simulink model "qpskTest"  (R2019b)
settings: Solver=VariableStepAuto  StartTime=0.0  StopTime=0.08  RelTol=1e-3
undefined symbols (not defined in the file): doppler, rsgenpoly
libraries: dspobslib x46, dspindex x4, commdigbbndpm3 x4, commchan3 x2, dspxfrm3 x2, commblkcod2 x2, commseqgen2 x2, commutil2 x2, commrandsrc2 x1, dspsigops x1, commsink2 x1
settings Model: Creator=mgege007  LastModifiedBy=mgege007

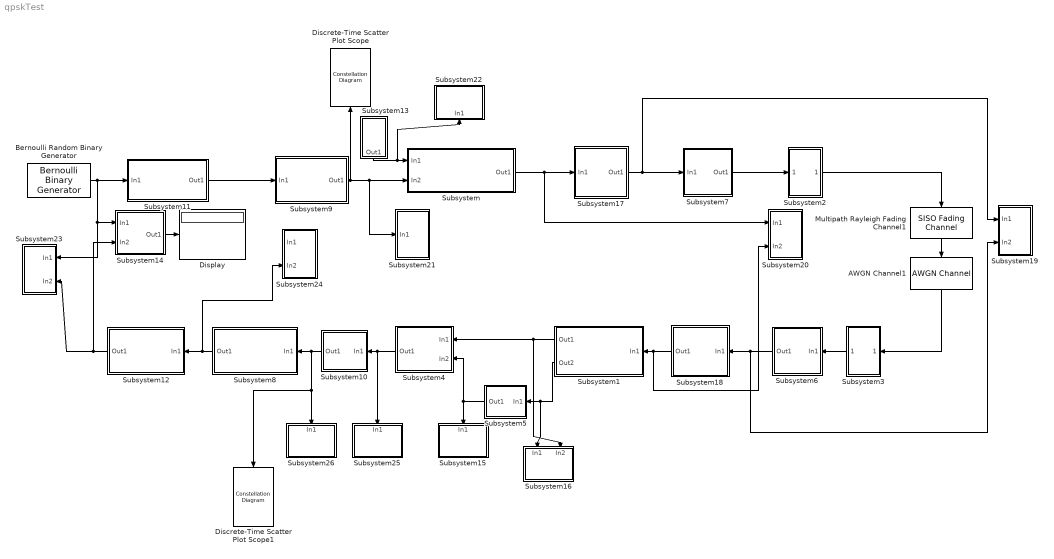
== system qpskTest ==
  AWGN Channel1 : commchan3/AWGN Channel  InputProcessing=Columns as channels (frame based)  seed=32965  noiseMode="Signal to noise ratio  (SNR)"  EbNodB=10  EsNodB=28  SNRdB=-15  bitsPerSym=1  Ps=30/(5.5e5*11/15*2.4)*1.08  Tsym=80e-6  variance=1
      settings: SourceProductName=Communications Toolbox
  Bernoulli Random Binary Generator : commrandsrc2/Bernoulli Binary Generator  P=[0.5]  seed=9364248  Ts=16e-5/44/2  frameBased=on  sampPerFrame=44  orient=off  outDataType=double
      settings: SourceProductName=Communications Toolbox  SourceProductBaseCode=CM
  Discrete-Time Scatter Plot Scope : ConstellationDiagram  Tag=ScatterPlot
  Discrete-Time Scatter Plot Scope1 : ConstellationDiagram  Tag=ScatterPlot
  Display : Display
  Multipath Rayleigh Fading Channel1 : commchan3/SISO Fading Channel  InheritSampleRate=on  SampleRate=1  PathDelays=[0 2e-6]  AveragePathGains=[0 -12]  NormalizePathGains=on  FadingDistribution=Rayleigh  KFactor=3  DirectPathDopplerShift=0  DirectPathInitialPhase=0  MaximumDopplerShift=40  DopplerSpectrum=doppler('Jakes')  RandomStream=mt19937ar with seed  Seed=73  PathGainsOutputPort=off  ChannelFilterDelayOutputPort=off  SimulateUsing=Interpreted execution  Visualization=Off  PathsForDopplerDisplay=1  SamplesToDisplay=25%
      settings: SourceProductName=Communications Toolbox
  Subsystem : Subsystem
      mask Display: disp('OFDM Baseband\nModulator\ndan\nAdd Cyclic Prefix')
  Subsystem1 : Subsystem
      mask Display: disp('OFDM Baseband\nDemodulator\ndan \nRemove Cyclic prefix')
  Subsystem10 : Subsystem
      mask Display: disp('Remove\nZero')
  Subsystem11 : Subsystem
      mask Display: disp('RS(15,11) Encoder')
  Subsystem12 : Subsystem
      mask Display: disp('RS(15,11) Decoder')
  Subsystem13 : Subsystem
      mask Display: disp('Training')
  Subsystem14 : Subsystem
      mask Display: disp('SER\nCalculation')
  Subsystem15 : Subsystem
  Subsystem16 : Subsystem
  Subsystem17 : Subsystem
      mask Display: disp('Add\nCyclic Prefix')
  Subsystem18 : Subsystem
      mask Display: disp('Remove\nCyclic Prefix')
  Subsystem19 : Subsystem
  Subsystem2 : Subsystem
      mask Display: disp('P/S')
  Subsystem20 : Subsystem
  Subsystem21 : Subsystem
  Subsystem22 : Subsystem
  Subsystem23 : Subsystem
  Subsystem24 : Subsystem
  Subsystem25 : Subsystem
  Subsystem26 : Subsystem
  Subsystem3 : Subsystem
      mask Display: disp('S/P')
  Subsystem4 : Subsystem
      mask Display: disp('Channel\nCompensation')
  Subsystem5 : Subsystem
      mask Display: disp('Channel\nEstimator')
  Subsystem6 : Subsystem
      mask Display: disp('Training\nSeparation')
  Subsystem7 : Subsystem
      mask Display: disp('Training\nInsertion')
  Subsystem8 : Subsystem
      mask Display: disp('QPSK Demapping')
  Subsystem9 : Subsystem
      mask Display: disp('QPSK Mapping')
  wires:
  Subsystem3/1(Out1) -> Subsystem6/1(In1)
  Subsystem17/1(Out1) -> Subsystem7/1(In1), Subsystem19/1(In1)
  Subsystem11/1(Out1) -> Subsystem9/1(In1)
  Subsystem13/1(Out1) -> Subsystem/1(In1), Subsystem22/1(In1)
  Subsystem6/1(Out1) -> Subsystem18/1(In1), Subsystem19/2(In2)
  Subsystem10/1(Out1) -> Subsystem8/1(In1), Subsystem26/1(In1), Discrete-Time Scatter Plot Scope1/1
  Bernoulli Random Binary Generator/1 -> Subsystem14/1(In1), Subsystem23/1(In1), Subsystem11/1(In1)
  Subsystem2/1(Out1) -> Multipath Rayleigh Fading Channel1/1
  Subsystem18/1(Out1) -> Subsystem1/1(In1), Subsystem20/2(In2)
  Subsystem14/1(Out1) -> Display/1
  Subsystem1/1(Out1) -> Subsystem4/1(In1), Subsystem16/2(In2)
  Multipath Rayleigh Fading Channel1/1 -> AWGN Channel1/1
  AWGN Channel1/1 -> Subsystem3/1(In1)
  Subsystem4/1(Out1) -> Subsystem10/1(In1), Subsystem25/1(In1)
  Subsystem7/1(Out1) -> Subsystem2/1(In1)
  Subsystem9/1(Out1) -> Subsystem/2(In2), Subsystem21/1(In1), Discrete-Time Scatter Plot Scope/1
  Subsystem5/1(Out1) -> Subsystem4/2(In2), Subsystem15/1(In1)
  Subsystem12/1(Out1) -> Subsystem14/2(In2), Subsystem23/2(In2)
  Subsystem1/2(Out2) -> Subsystem5/1(In1), Subsystem16/1(In1)
  Subsystem8/1(Out1) -> Subsystem12/1(In1), Subsystem24/2(In2)
  Subsystem/1(Out1) -> Subsystem17/1(In1), Subsystem20/1(In1)

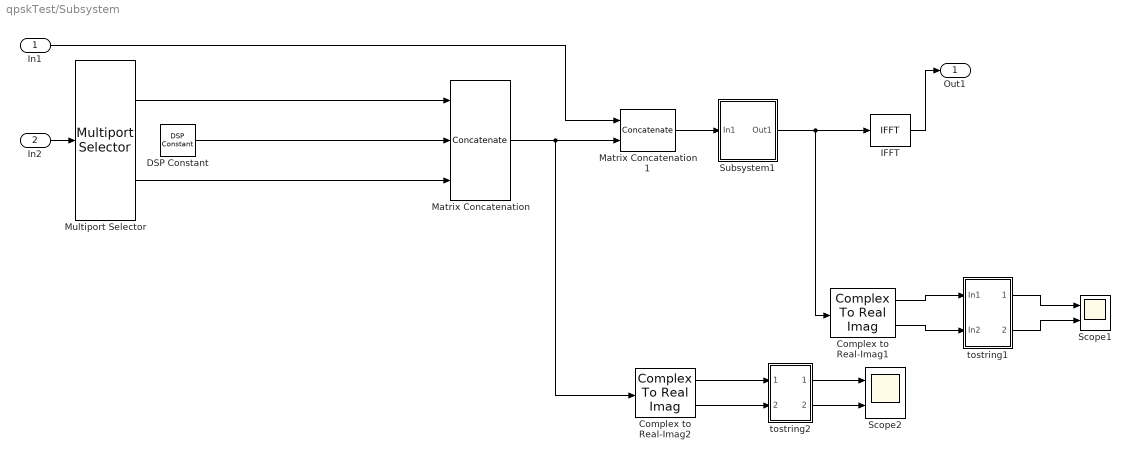
== system qpskTest/Subsystem ==
  In1 : Inport
  In2 : Inport  Port=2
  Complex to Real-Imag1 : ComplexToRealImag
  Complex to Real-Imag2 : ComplexToRealImag
  DSP Constant : dspobslib/DSP Constant  Value=0  SampleMode=Discrete  discreteOutput=Frame-based  continuousOutput=Sample-based  sampTime=16e-5/2  framePeriod=16e-5/2  dataType=Inherit from 'Constant value'  isSigned=on  wordLen=16  udDataType=sfix(16)  fracBitsMode=Best precision  numFracBits=15  InterpretAs1D=off  Ts=16e-5/2  FramebasedOutput=on
      settings: SourceProductName=DSP System Toolbox  SourceProductBaseCode=DS
  IFFT : dspxfrm3/IFFT  FFTImplementation=Auto  CompMethod=Table lookup  TableOpt=HYBRID  TableOptActive=Speed  BitRevOrder=off  cs_in=off  Normalize=on  InheritFFTLength=on  FFTLength=64  WrapInput=on  mode=Real  outSamplingMode=Frame based  roundingMode=Floor  overflowMode=off  firstCoeffDataTypeStr=Inherit: Same word length as input  firstCoeffLastDataTypeStr=Inherit: Same word length as input  outputMin=[]  outputMax=[]
      settings: SourceProductName=DSP System Toolbox
  Matrix Concatenation : Concatenate  NumInputs=3  Mode=Multidimensional array
  Matrix Concatenation1 : Concatenate  Mode=Multidimensional array  ConcatenateDimension=2
  Multiport Selector : dspindex/Multiport Selector  rowsOrCols=Rows  idxCellArray={1:15,16:30}  idxErrMode=Clip Index
  Scope1 : Scope  NumInputPorts=2
  Scope2 : Scope  NumInputPorts=2
  Subsystem1 : Subsystem
      mask Display: disp('Zero Pad')
  tostring1 : Subsystem
  tostring2 : Subsystem
  Out1 : Outport
  wires:
  IFFT/1 -> Out1/1
  Multiport Selector/1 -> Matrix Concatenation/1
  Multiport Selector/2 -> Matrix Concatenation/3
  DSP Constant/1 -> Matrix Concatenation/2
  Subsystem1/1(Out1) -> IFFT/1, Complex to Real-Imag1/1
  In2/1 -> Multiport Selector/1
  Matrix Concatenation1/1 -> Subsystem1/1(In1)
  Matrix Concatenation/1 -> Matrix Concatenation1/2, Complex to Real-Imag2/1
  In1/1 -> Matrix Concatenation1/1
  Complex to Real-Imag1/1 -> tostring1/1(In1)
  Complex to Real-Imag1/2 -> tostring1/2(In2)
  tostring1/1(Out1) -> Scope1/1
  tostring1/2(Out2) -> Scope1/2
  Complex to Real-Imag2/1 -> tostring2/1(In1)
  Complex to Real-Imag2/2 -> tostring2/2(In2)
  tostring2/1(Out1) -> Scope2/1
  tostring2/2(Out2) -> Scope2/2

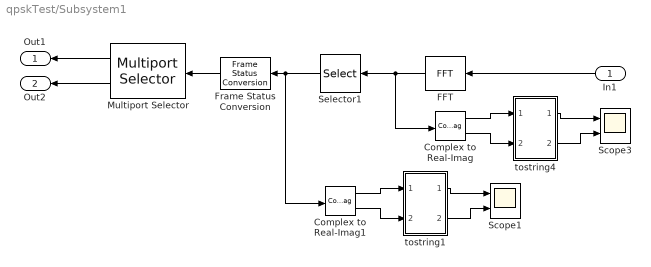
== system qpskTest/Subsystem1 ==
  In1 : Inport
  Complex to Real-Imag : ComplexToRealImag
  Complex to Real-Imag1 : ComplexToRealImag
  FFT : dspxfrm3/FFT  FFTImplementation=Auto  CompMethod=Table lookup  TableOpt=HYBRID  TableOptActive=Speed  BitRevOrder=off  Normalize=off  InheritFFTLength=on  FFTLength=64  WrapInput=on  roundingMode=Floor  overflowMode=off  firstCoeffDataTypeStr=Inherit: Same word length as input  firstCoeffLastDataTypeStr=Inherit: Same word length as input  outputMin=[]  outputMax=[]
  Frame Status Conversion : dspobslib/Frame Status Conversion  growRefPort=off  outframe=Frame-based
      settings: SourceProductName=DSP System Toolbox  SourceProductBaseCode=DS
  Multiport Selector : dspindex/Multiport Selector  rowsOrCols=Columns  idxCellArray={1,2}  idxErrMode=Clip Index
  Scope1 : Scope  NumInputPorts=2
  Scope3 : Scope  NumInputPorts=2
  Selector1 : Selector  NumberOfDimensions=2  InputPortWidth=64  IndexOptions=Index vector (dialog),Select all  Indices=[50:64,1:16],-1  OutputSizes=1
  tostring1 : Subsystem
  tostring4 : Subsystem
  Out1 : Outport
  Out2 : Outport  Port=2
  wires:
  FFT/1 -> Selector1/1, Complex to Real-Imag/1
  Selector1/1 -> Frame Status Conversion/1, Complex to Real-Imag1/1
  In1/1 -> FFT/1
  Frame Status Conversion/1 -> Multiport Selector/1
  Multiport Selector/1 -> Out1/1
  Multiport Selector/2 -> Out2/1
  Complex to Real-Imag/1 -> tostring4/1(In1)
  Complex to Real-Imag/2 -> tostring4/2(In2)
  tostring4/1(Out1) -> Scope3/1
  tostring4/2(Out2) -> Scope3/2
  Complex to Real-Imag1/1 -> tostring1/1(In1)
  Complex to Real-Imag1/2 -> tostring1/2(In2)
  tostring1/1(Out1) -> Scope1/1
  tostring1/2(Out2) -> Scope1/2

== system qpskTest/Subsystem10 ==
  In1 : Inport
  Selector2 : Selector  NumberOfDimensions=2  InputPortWidth=31  IndexOptions=Index vector (dialog),Select all  Indices=[1:15,17:31],-1  OutputSizes=1
  Out1 : Outport
  wires:
  Selector2/1 -> Out1/1
  In1/1 -> Selector2/1

== system qpskTest/Subsystem11 ==
  In1 : Inport
  Binary-Input RS Encoder : commblkcod2/Binary-Input RS Encoder  n=15  k=11  specShortening=off  shortenedK=3  specGenPoly=off  genPoly=rsgenpoly(7,3)  specPrimPoly=off  prPoly=[1 0 1 1]  specPuncture=off  punctVec=[ones(2,1); zeros(2,1)]  outDType=Same as input
      settings: SourceProductName=Communications Toolbox  SourceProductBaseCode=CM
  Out1 : Outport
  wires:
  In1/1 -> Binary-Input RS Encoder/1
  Binary-Input RS Encoder/1 -> Out1/1

== system qpskTest/Subsystem12 ==
  In1 : Inport
  Binary-Output RS Decoder : commblkcod2/Binary-Output RS Decoder  n=15  k=11  specShortening=off  shortenedK=3  specGenPoly=off  genPoly=rsgenpoly(7,3)  specPrimPoly=off  prPoly=[1 0 1 1]  specPuncture=off  punctVec=[ones(2,1); zeros(2,1)]  specErasurePort=off  showNumErr=on  outDType=Same as input
      settings: SourceProductName=Communications Toolbox  SourceProductBaseCode=CM
  Terminator : Terminator
  Out1 : Outport
  wires:
  Binary-Output RS Decoder/2 -> Terminator/1
  Binary-Output RS Decoder/1 -> Out1/1
  In1/1 -> Binary-Output RS Decoder/1

== system qpskTest/Subsystem13 ==
  PN Sequence Generator : commseqgen2/PN Sequence Generator  poly=[1 0 0 0 0 1 1]  ini_sta=[0 0 0 0 0 1]  outBitMaskSource=Dialog parameter  shift=0  outVarSiz=off  maxOutSizeMode=Dialog parameter  maxOutSize=[10 1]  Ts=16e-5/2/31  frameBased=on  sampPerFrame=31  reset=off  bitPackedOutputs=off  outDataType=double  numPackedBits=8  bitPackDataSigned=off  bitPackedOutDType=double
      settings: SourceProductName=Communications Toolbox  SourceProductBaseCode=CM
  Unipolar to Bipolar Converter : commutil2/Unipolar to Bipolar Converter  M=2  polarity=Positive  dataType=Inherit via internal rule
      settings: SourceProductName=Communications Toolbox
  Out1 : Outport
  wires:
  PN Sequence Generator/1 -> Unipolar to Bipolar Converter/1
  Unipolar to Bipolar Converter/1 -> Out1/1

== system qpskTest/Subsystem14 ==
  In1 : Inport
  In2 : Inport  Port=2
  Error Rate Calculation : commsink2/Error Rate Calculation  N=22  st_delay=0  cp_mode=Entire frame  subframe=[]  PMode=Port  WsName=ErrorVec  RsMode2=off  stop=off  numErr=inf  maxBits=2e4
      settings: SourceProductName=Communications Toolbox
  QPSK Modulator Baseband : commdigbbndpm3/QPSK Modulator Baseband  InType=Bit  Enc=Binary  Ph=pi/4  outDtype=double  outWordLen=16  outUDDataType=sfix(16)  outFracLenMode=Best precision  outFracLen=15  outDataTypeStr=double  outLastDataTypeStr=double
      settings: SourceProductName=Communications Toolbox
  QPSK Modulator Baseband1 : commdigbbndpm3/QPSK Modulator Baseband  InType=Bit  Enc=Binary  Ph=pi/4  outDtype=double  outWordLen=16  outUDDataType=sfix(16)  outFracLenMode=Best precision  outFracLen=15  outDataTypeStr=double  outLastDataTypeStr=double
      settings: SourceProductName=Communications Toolbox
  Out1 : Outport
  wires:
  QPSK Modulator Baseband/1 -> Error Rate Calculation/1
  QPSK Modulator Baseband1/1 -> Error Rate Calculation/2
  In1/1 -> QPSK Modulator Baseband/1
  Error Rate Calculation/1 -> Out1/1
  In2/1 -> QPSK Modulator Baseband1/1

== system qpskTest/Subsystem15 ==
  In1 : Inport
  Complex to Real-Imag7 : ComplexToRealImag
  Scope7 : Scope  NumInputPorts=2
  tostring9 : Subsystem
  wires:
  Complex to Real-Imag7/1 -> tostring9/1(In1)
  Complex to Real-Imag7/2 -> tostring9/2(In2)
  tostring9/1(Out1) -> Scope7/1
  tostring9/2(Out2) -> Scope7/2
  In1/1 -> Complex to Real-Imag7/1

== system qpskTest/Subsystem16 ==
  In1 : Inport
  In2 : Inport  Port=2
  Complex to Real-Imag5 : ComplexToRealImag
  Complex to Real-Imag6 : ComplexToRealImag
  Scope6 : Scope  NumInputPorts=4
  tostring8 : Subsystem
  wires:
  tostring8/1(Out1) -> Scope6/1
  tostring8/2(Out2) -> Scope6/2
  Complex to Real-Imag5/1 -> tostring8/1(In1)
  Complex to Real-Imag5/2 -> tostring8/2(In2)
  Complex to Real-Imag6/1 -> tostring8/3(In3)
  Complex to Real-Imag6/2 -> tostring8/4(In4)
  tostring8/3(Out3) -> Scope6/3
  tostring8/4(Out4) -> Scope6/4
  In1/1 -> Complex to Real-Imag5/1
  In2/1 -> Complex to Real-Imag6/1

== system qpskTest/Subsystem17 ==
  In1 : Inport
  Selector3 : Selector  NumberOfDimensions=2  InputPortWidth=64  IndexOptions=Index vector (dialog),Select all  Indices=[39:64,1:64],-1  OutputSizes=1
  Out1 : Outport
  wires:
  Selector3/1 -> Out1/1
  In1/1 -> Selector3/1

== system qpskTest/Subsystem18 ==
  In1 : Inport
  Selector4 : Selector  NumberOfDimensions=2  InputPortWidth=78  IndexOptions=Index vector (dialog),Select all  Indices=[27:90],-1  OutputSizes=1
  Out1 : Outport
  wires:
  Selector4/1 -> Out1/1
  In1/1 -> Selector4/1

== system qpskTest/Subsystem19 ==
  In1 : Inport
  In2 : Inport  Port=2
  Complex to Real-Imag1 : ComplexToRealImag
  Complex to Real-Imag2 : ComplexToRealImag
  Scope4 : Scope  NumInputPorts=4
  tostring5 : Subsystem
  tostring6 : Subsystem
  wires:
  Complex to Real-Imag1/1 -> tostring5/1(In1)
  Complex to Real-Imag1/2 -> tostring5/2(In2)
  tostring5/1(Out1) -> Scope4/1
  Complex to Real-Imag2/1 -> tostring6/1(In1)
  Complex to Real-Imag2/2 -> tostring6/2(In2)
  tostring6/1(Out1) -> Scope4/2
  tostring5/2(Out2) -> Scope4/3
  tostring6/2(Out2) -> Scope4/4
  In1/1 -> Complex to Real-Imag1/1
  In2/1 -> Complex to Real-Imag2/1

== system qpskTest/Subsystem2 ==
  In1 : Inport
  Unbuffer3 : Unbuffer
  Out1 : Outport
  wires:
  In1/1 -> Unbuffer3/1
  Unbuffer3/1 -> Out1/1

== system qpskTest/Subsystem20 ==
  In1 : Inport
  In2 : Inport  Port=2
  Complex to Real-Imag3 : ComplexToRealImag
  Complex to Real-Imag4 : ComplexToRealImag
  Scope5 : Scope  NumInputPorts=4
  tostring7 : Subsystem
  wires:
  Complex to Real-Imag3/1 -> tostring7/1(In1)
  Complex to Real-Imag3/2 -> tostring7/2(In2)
  tostring7/1(Out1) -> Scope5/1
  Complex to Real-Imag4/1 -> tostring7/3(In3)
  Complex to Real-Imag4/2 -> tostring7/4(In4)
  tostring7/3(Out3) -> Scope5/2
  tostring7/2(Out2) -> Scope5/3
  tostring7/4(Out4) -> Scope5/4
  In1/1 -> Complex to Real-Imag3/1
  In2/1 -> Complex to Real-Imag4/1

== system qpskTest/Subsystem21 ==
  In1 : Inport
  Complex to Real-Imag : ComplexToRealImag
  Scope3 : Scope  NumInputPorts=2
  tostring4 : Subsystem
  wires:
  Complex to Real-Imag/1 -> tostring4/1(In1)
  Complex to Real-Imag/2 -> tostring4/2(In2)
  tostring4/1(Out1) -> Scope3/1
  tostring4/2(Out2) -> Scope3/2
  In1/1 -> Complex to Real-Imag/1

== system qpskTest/Subsystem22 ==
  In1 : Inport
  Scope2 : Scope
  tostring3 : Subsystem
  wires:
  tostring3/1(Out1) -> Scope2/1
  In1/1 -> tostring3/1(In1)

== system qpskTest/Subsystem23 ==
  In1 : Inport
  In2 : Inport  Port=2
  Scope : Scope  NumInputPorts=2
  tostring : Subsystem
  tostring1 : Subsystem
  wires:
  tostring/1(Out1) -> Scope/1
  tostring1/1(Out1) -> Scope/2
  In1/1 -> tostring/1(In1)
  In2/1 -> tostring1/1(In1)

== system qpskTest/Subsystem24 ==
  In1 : Inport
  In2 : Inport  Port=2
  Scope1 : Scope  NumInputPorts=2
  tostring2 : Subsystem
  wires:
  tostring2/1(Out1) -> Scope1/1
  tostring2/2(Out2) -> Scope1/2
  In1/1 -> tostring2/1(In1)
  In2/1 -> tostring2/2(In2)

== system qpskTest/Subsystem25 ==
  In1 : Inport
  Complex to Real-Imag7 : ComplexToRealImag
  Scope7 : Scope  NumInputPorts=2
  tostring9 : Subsystem
  wires:
  Complex to Real-Imag7/1 -> tostring9/1(In1)
  Complex to Real-Imag7/2 -> tostring9/2(In2)
  tostring9/1(Out1) -> Scope7/1
  tostring9/2(Out2) -> Scope7/2
  In1/1 -> Complex to Real-Imag7/1

== system qpskTest/Subsystem26 ==
  In1 : Inport
  Complex to Real-Imag7 : ComplexToRealImag
  Scope7 : Scope  NumInputPorts=2
  tostring9 : Subsystem
  wires:
  Complex to Real-Imag7/1 -> tostring9/1(In1)
  Complex to Real-Imag7/2 -> tostring9/2(In2)
  tostring9/1(Out1) -> Scope7/1
  tostring9/2(Out2) -> Scope7/2
  In1/1 -> Complex to Real-Imag7/1

== system qpskTest/Subsystem3 ==
  In1 : Inport
  Buffer : Buffer  N=180
  Out1 : Outport
  wires:
  In1/1 -> Buffer/1
  Buffer/1 -> Out1/1

== system qpskTest/Subsystem4 ==
  In1 : Inport
  In2 : Inport  Port=2
  Frame Status Conversion5 : dspobslib/Frame Status Conversion  growRefPort=off  outframe=Frame-based
      settings: SourceProductName=DSP System Toolbox  SourceProductBaseCode=DS
  Product : Product  SaturateOnIntegerOverflow=on  OutDataTypeStr=Inherit: Same as first input
  Out1 : Outport
  wires:
  Frame Status Conversion5/1 -> Out1/1
  In2/1 -> Product/1
  Product/1 -> Frame Status Conversion5/1
  In1/1 -> Product/2

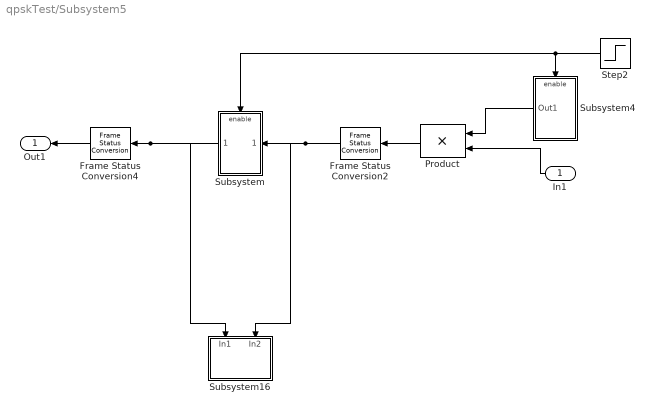
== system qpskTest/Subsystem5 ==
  In1 : Inport
  Frame Status Conversion2 : dspobslib/Frame Status Conversion  growRefPort=off  outframe=Frame-based
      settings: SourceProductName=DSP System Toolbox  SourceProductBaseCode=DS
  Frame Status Conversion4 : dspobslib/Frame Status Conversion  growRefPort=off  outframe=Frame-based
      settings: SourceProductName=DSP System Toolbox  SourceProductBaseCode=DS
  Product : Product  SaturateOnIntegerOverflow=on  OutDataTypeStr=Inherit: Same as first input
  Step2 : Step  Time=16e-5/2  SampleTime=16e-5/2
  Subsystem : Subsystem
  Subsystem16 : Subsystem
  Subsystem4 : Subsystem  TreatAsAtomicUnit=on
  Out1 : Outport
  wires:
  Step2/1 -> Subsystem4/Enable, Subsystem/Enable
  Subsystem4/1(Out1) -> Product/1
  Product/1 -> Frame Status Conversion2/1
  Frame Status Conversion2/1 -> Subsystem/1(In1), Subsystem16/2(In2)
  Frame Status Conversion4/1 -> Out1/1
  In1/1 -> Product/2
  Subsystem/1(Out1) -> Frame Status Conversion4/1, Subsystem16/1(In1)

== system qpskTest/Subsystem6 ==
  In1 : Inport
  Matrix Concatenation1 : Concatenate  Mode=Multidimensional array  ConcatenateDimension=2
  Multiport Selector1 : dspindex/Multiport Selector  rowsOrCols=Rows  idxCellArray={91:180,1:90}  idxErrMode=Clip Index
  Out1 : Outport
  wires:
  Multiport Selector1/2 -> Matrix Concatenation1/2
  Multiport Selector1/1 -> Matrix Concatenation1/1
  In1/1 -> Multiport Selector1/1
  Matrix Concatenation1/1 -> Out1/1

== system qpskTest/Subsystem7 ==
  In1 : Inport
  Frame Status Conversion : dspobslib/Frame Status Conversion  growRefPort=off  outframe=Frame-based
      settings: SourceProductName=DSP System Toolbox  SourceProductBaseCode=DS
  Matrix Concatenation : Concatenate  Mode=Multidimensional array
  Multiport Selector : dspindex/Multiport Selector  rowsOrCols=Columns  idxCellArray={1,2}  idxErrMode=Clip Index
  Out1 : Outport
  wires:
  Multiport Selector/1 -> Matrix Concatenation/1
  Multiport Selector/2 -> Matrix Concatenation/2
  Matrix Concatenation/1 -> Frame Status Conversion/1
  In1/1 -> Multiport Selector/1
  Frame Status Conversion/1 -> Out1/1

== system qpskTest/Subsystem8 ==
  In1 : Inport
  Gain : Gain  Gain=0.75  SaturateOnIntegerOverflow=on  OutDataTypeStr=Inherit: Same as input  ParamDataTypeStr=Inherit: Same as input
  QPSK Demodulator Baseband : commdigbbndpm3/QPSK Demodulator Baseband  OutType=Bit  DecType=Hard decision  VarSource=Dialog  Variance=1  Dec=Binary  Ph=pi/4  outDtype1=Inherit via internal rule  outDtype2=Inherit via internal rule  derotateFactorWordLen=16  derotateFactorDataTypeStr=Inherit: Same word length as input  derotateFactorLastDataTypeStr=Inherit: Same word length as input
      settings: SourceProductName=Communications Toolbox
  Rounding Function : Rounding  Operator=round
  Out1 : Outport
  wires:
  In1/1 -> Gain/1
  Rounding Function/1 -> Out1/1
  QPSK Demodulator Baseband/1 -> Rounding Function/1
  Gain/1 -> QPSK Demodulator Baseband/1

== system qpskTest/Subsystem9 ==
  In1 : Inport
  Gain : Gain  Gain=1/0.75  SaturateOnIntegerOverflow=on  OutDataTypeStr=Inherit: Same as input  ParamDataTypeStr=Inherit: Same as input
  QPSK Modulator Baseband : commdigbbndpm3/QPSK Modulator Baseband  InType=Bit  Enc=Binary  Ph=pi/4  outDtype=double  outWordLen=16  outUDDataType=sfix(16)  outFracLenMode=Best precision  outFracLen=15  outDataTypeStr=double  outLastDataTypeStr=double
      settings: SourceProductName=Communications Toolbox
  Out1 : Outport
  wires:
  QPSK Modulator Baseband/1 -> Gain/1
  In1/1 -> QPSK Modulator Baseband/1
  Gain/1 -> Out1/1

== system qpskTest/Subsystem/Subsystem1 ==
  In1 : Inport
  Selector : Selector  NumberOfDimensions=2  InputPortWidth=64  IndexOptions=Index vector (dialog),Select all  Indices=[16:64,1:15],-1  OutputSizes=1
  Zero Pad : dspsigops/Pad  padAlong=Columns and rows  dimsToPad=1  valSrc=Specify via dialog  padVal=0  spec=Output size  padNumOutRowsSpecMethod=User-specified  numOutRows=64  padNumOutColsSpecMethod=User-specified  numOutCols=2  isVarDimsMode=off  padBeginning=0  padEnd=0  outSizeMode=User-specified  outSize=1  padSigAt=End  trunc_flag=None  roundingMode=Floor  overflowMode=off  truncOrWrapMode=Truncate  wrap_flag=None
      settings: SourceProductName=DSP System Toolbox  SourceProductBaseCode=DS
  Out1 : Outport
  wires:
  Zero Pad/1 -> Selector/1
  In1/1 -> Zero Pad/1
  Selector/1 -> Out1/1

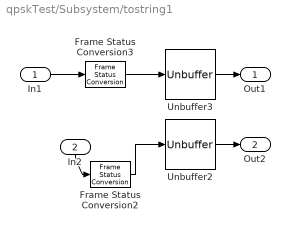
== system qpskTest/Subsystem/tostring1 ==
  In1 : Inport
  In2 : Inport  Port=2
  Frame Status Conversion2 : dspobslib/Frame Status Conversion  growRefPort=off  outframe=Sample-based
      settings: SourceProductName=DSP System Toolbox  SourceProductBaseCode=DS
  Frame Status Conversion3 : dspobslib/Frame Status Conversion  growRefPort=off  outframe=Sample-based
      settings: SourceProductName=DSP System Toolbox  SourceProductBaseCode=DS
  Unbuffer2 : Unbuffer
  Unbuffer3 : Unbuffer
  Out1 : Outport
  Out2 : Outport  Port=2
  wires:
  Frame Status Conversion3/1 -> Unbuffer3/1
  Frame Status Conversion2/1 -> Unbuffer2/1
  In1/1 -> Frame Status Conversion3/1
  In2/1 -> Frame Status Conversion2/1
  Unbuffer3/1 -> Out1/1
  Unbuffer2/1 -> Out2/1

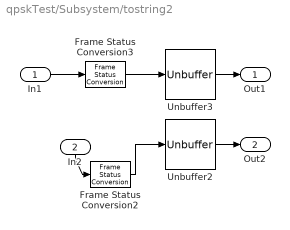
== system qpskTest/Subsystem/tostring2 ==
  In1 : Inport
  In2 : Inport  Port=2
  Frame Status Conversion2 : dspobslib/Frame Status Conversion  growRefPort=off  outframe=Sample-based
      settings: SourceProductName=DSP System Toolbox  SourceProductBaseCode=DS
  Frame Status Conversion3 : dspobslib/Frame Status Conversion  growRefPort=off  outframe=Sample-based
      settings: SourceProductName=DSP System Toolbox  SourceProductBaseCode=DS
  Unbuffer2 : Unbuffer
  Unbuffer3 : Unbuffer
  Out1 : Outport
  Out2 : Outport  Port=2
  wires:
  Frame Status Conversion3/1 -> Unbuffer3/1
  Frame Status Conversion2/1 -> Unbuffer2/1
  In1/1 -> Frame Status Conversion3/1
  In2/1 -> Frame Status Conversion2/1
  Unbuffer3/1 -> Out1/1
  Unbuffer2/1 -> Out2/1

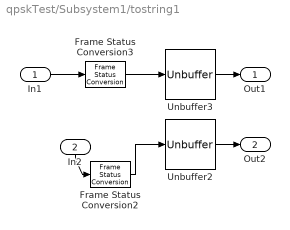
== system qpskTest/Subsystem1/tostring1 ==
  In1 : Inport
  In2 : Inport  Port=2
  Frame Status Conversion2 : dspobslib/Frame Status Conversion  growRefPort=off  outframe=Sample-based
      settings: SourceProductName=DSP System Toolbox  SourceProductBaseCode=DS
  Frame Status Conversion3 : dspobslib/Frame Status Conversion  growRefPort=off  outframe=Sample-based
      settings: SourceProductName=DSP System Toolbox  SourceProductBaseCode=DS
  Unbuffer2 : Unbuffer
  Unbuffer3 : Unbuffer
  Out1 : Outport
  Out2 : Outport  Port=2
  wires:
  Frame Status Conversion3/1 -> Unbuffer3/1
  Frame Status Conversion2/1 -> Unbuffer2/1
  In1/1 -> Frame Status Conversion3/1
  In2/1 -> Frame Status Conversion2/1
  Unbuffer3/1 -> Out1/1
  Unbuffer2/1 -> Out2/1

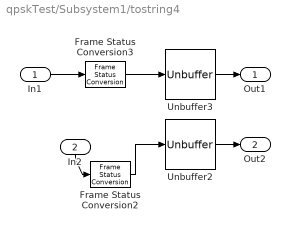
== system qpskTest/Subsystem1/tostring4 ==
  In1 : Inport
  In2 : Inport  Port=2
  Frame Status Conversion2 : dspobslib/Frame Status Conversion  growRefPort=off  outframe=Sample-based
      settings: SourceProductName=DSP System Toolbox  SourceProductBaseCode=DS
  Frame Status Conversion3 : dspobslib/Frame Status Conversion  growRefPort=off  outframe=Sample-based
      settings: SourceProductName=DSP System Toolbox  SourceProductBaseCode=DS
  Unbuffer2 : Unbuffer
  Unbuffer3 : Unbuffer
  Out1 : Outport
  Out2 : Outport  Port=2
  wires:
  Frame Status Conversion3/1 -> Unbuffer3/1
  Frame Status Conversion2/1 -> Unbuffer2/1
  In1/1 -> Frame Status Conversion3/1
  In2/1 -> Frame Status Conversion2/1
  Unbuffer3/1 -> Out1/1
  Unbuffer2/1 -> Out2/1

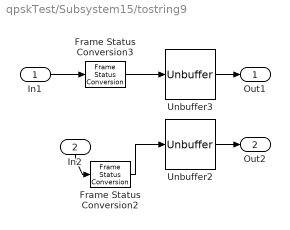
== system qpskTest/Subsystem15/tostring9 ==
  In1 : Inport
  In2 : Inport  Port=2
  Frame Status Conversion2 : dspobslib/Frame Status Conversion  growRefPort=off  outframe=Sample-based
      settings: SourceProductName=DSP System Toolbox  SourceProductBaseCode=DS
  Frame Status Conversion3 : dspobslib/Frame Status Conversion  growRefPort=off  outframe=Sample-based
      settings: SourceProductName=DSP System Toolbox  SourceProductBaseCode=DS
  Unbuffer2 : Unbuffer
  Unbuffer3 : Unbuffer
  Out1 : Outport
  Out2 : Outport  Port=2
  wires:
  Frame Status Conversion3/1 -> Unbuffer3/1
  Frame Status Conversion2/1 -> Unbuffer2/1
  In1/1 -> Frame Status Conversion3/1
  In2/1 -> Frame Status Conversion2/1
  Unbuffer3/1 -> Out1/1
  Unbuffer2/1 -> Out2/1

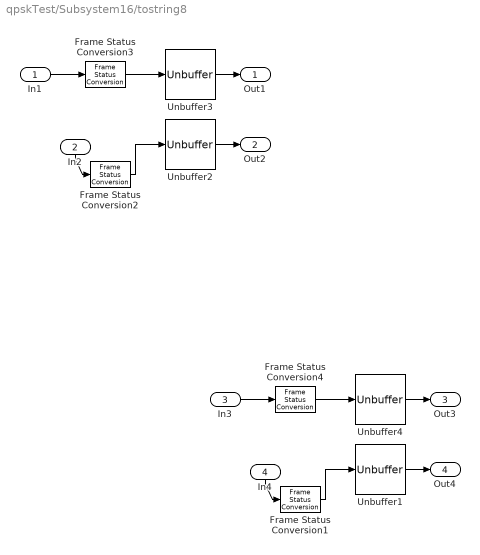
== system qpskTest/Subsystem16/tostring8 ==
  In1 : Inport
  In2 : Inport  Port=2
  In3 : Inport  Port=3
  In4 : Inport  Port=4
  Frame Status Conversion{1..4} (4 alike) : dspobslib/Frame Status Conversion  growRefPort=off  outframe=Sample-based
      settings: SourceProductName=DSP System Toolbox  SourceProductBaseCode=DS
  Unbuffer{1..4} (4 alike) : Unbuffer
  Out1 : Outport
  Out2 : Outport  Port=2
  Out3 : Outport  Port=3
  Out4 : Outport  Port=4
  wires:
  Frame Status Conversion3/1 -> Unbuffer3/1
  Frame Status Conversion2/1 -> Unbuffer2/1
  In1/1 -> Frame Status Conversion3/1
  In2/1 -> Frame Status Conversion2/1
  Unbuffer3/1 -> Out1/1
  Unbuffer2/1 -> Out2/1
  Frame Status Conversion4/1 -> Unbuffer4/1
  Frame Status Conversion1/1 -> Unbuffer1/1
  In3/1 -> Frame Status Conversion4/1
  In4/1 -> Frame Status Conversion1/1
  Unbuffer4/1 -> Out3/1
  Unbuffer1/1 -> Out4/1

== system qpskTest/Subsystem19/tostring5 ==
  In1 : Inport
  In2 : Inport  Port=2
  Frame Status Conversion2 : dspobslib/Frame Status Conversion  growRefPort=off  outframe=Sample-based
      settings: SourceProductName=DSP System Toolbox  SourceProductBaseCode=DS
  Frame Status Conversion3 : dspobslib/Frame Status Conversion  growRefPort=off  outframe=Sample-based
      settings: SourceProductName=DSP System Toolbox  SourceProductBaseCode=DS
  Unbuffer2 : Unbuffer
  Unbuffer3 : Unbuffer
  Out1 : Outport
  Out2 : Outport  Port=2
  wires:
  Frame Status Conversion3/1 -> Unbuffer3/1
  Frame Status Conversion2/1 -> Unbuffer2/1
  In1/1 -> Frame Status Conversion3/1
  In2/1 -> Frame Status Conversion2/1
  Unbuffer3/1 -> Out1/1
  Unbuffer2/1 -> Out2/1

== system qpskTest/Subsystem19/tostring6 ==
  In1 : Inport
  In2 : Inport  Port=2
  Frame Status Conversion2 : dspobslib/Frame Status Conversion  growRefPort=off  outframe=Sample-based
      settings: SourceProductName=DSP System Toolbox  SourceProductBaseCode=DS
  Frame Status Conversion3 : dspobslib/Frame Status Conversion  growRefPort=off  outframe=Sample-based
      settings: SourceProductName=DSP System Toolbox  SourceProductBaseCode=DS
  Unbuffer2 : Unbuffer
  Unbuffer3 : Unbuffer
  Out1 : Outport
  Out2 : Outport  Port=2
  wires:
  Frame Status Conversion3/1 -> Unbuffer3/1
  Frame Status Conversion2/1 -> Unbuffer2/1
  In1/1 -> Frame Status Conversion3/1
  In2/1 -> Frame Status Conversion2/1
  Unbuffer3/1 -> Out1/1
  Unbuffer2/1 -> Out2/1

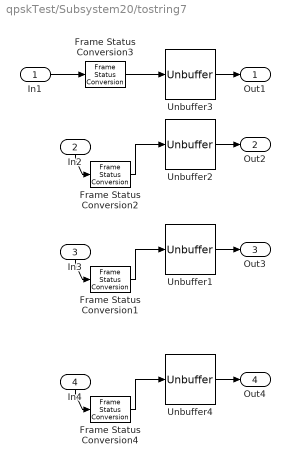
== system qpskTest/Subsystem20/tostring7 ==
  In1 : Inport
  In2 : Inport  Port=2
  In3 : Inport  Port=3
  In4 : Inport  Port=4
  Frame Status Conversion{1..4} (4 alike) : dspobslib/Frame Status Conversion  growRefPort=off  outframe=Sample-based
      settings: SourceProductName=DSP System Toolbox  SourceProductBaseCode=DS
  Unbuffer{1..4} (4 alike) : Unbuffer
  Out1 : Outport
  Out2 : Outport  Port=2
  Out3 : Outport  Port=3
  Out4 : Outport  Port=4
  wires:
  Frame Status Conversion3/1 -> Unbuffer3/1
  Frame Status Conversion2/1 -> Unbuffer2/1
  In1/1 -> Frame Status Conversion3/1
  In2/1 -> Frame Status Conversion2/1
  Unbuffer3/1 -> Out1/1
  Unbuffer2/1 -> Out2/1
  Frame Status Conversion1/1 -> Unbuffer1/1
  In3/1 -> Frame Status Conversion1/1
  Unbuffer1/1 -> Out3/1
  Frame Status Conversion4/1 -> Unbuffer4/1
  In4/1 -> Frame Status Conversion4/1
  Unbuffer4/1 -> Out4/1

== system qpskTest/Subsystem21/tostring4 ==
  In1 : Inport
  In2 : Inport  Port=2
  Frame Status Conversion2 : dspobslib/Frame Status Conversion  growRefPort=off  outframe=Sample-based
      settings: SourceProductName=DSP System Toolbox  SourceProductBaseCode=DS
  Frame Status Conversion3 : dspobslib/Frame Status Conversion  growRefPort=off  outframe=Sample-based
      settings: SourceProductName=DSP System Toolbox  SourceProductBaseCode=DS
  Unbuffer2 : Unbuffer
  Unbuffer3 : Unbuffer
  Out1 : Outport
  Out2 : Outport  Port=2
  wires:
  Frame Status Conversion3/1 -> Unbuffer3/1
  Frame Status Conversion2/1 -> Unbuffer2/1
  In1/1 -> Frame Status Conversion3/1
  In2/1 -> Frame Status Conversion2/1
  Unbuffer3/1 -> Out1/1
  Unbuffer2/1 -> Out2/1

== system qpskTest/Subsystem22/tostring3 ==
  In1 : Inport
  Frame Status Conversion1 : dspobslib/Frame Status Conversion  growRefPort=off  outframe=Sample-based
      settings: SourceProductName=DSP System Toolbox  SourceProductBaseCode=DS
  Unbuffer1 : Unbuffer
  Out1 : Outport
  wires:
  Frame Status Conversion1/1 -> Unbuffer1/1
  In1/1 -> Frame Status Conversion1/1
  Unbuffer1/1 -> Out1/1

== system qpskTest/Subsystem23/tostring ==
  In1 : Inport
  Frame Status Conversion5 : dspobslib/Frame Status Conversion  growRefPort=off  outframe=Sample-based
      settings: SourceProductName=DSP System Toolbox  SourceProductBaseCode=DS
  Unbuffer : Unbuffer
  Out1 : Outport
  wires:
  Frame Status Conversion5/1 -> Unbuffer/1
  In1/1 -> Frame Status Conversion5/1
  Unbuffer/1 -> Out1/1

== system qpskTest/Subsystem23/tostring1 ==
  In1 : Inport
  Frame Status Conversion1 : dspobslib/Frame Status Conversion  growRefPort=off  outframe=Sample-based
      settings: SourceProductName=DSP System Toolbox  SourceProductBaseCode=DS
  Unbuffer1 : Unbuffer
  Out1 : Outport
  wires:
  Frame Status Conversion1/1 -> Unbuffer1/1
  In1/1 -> Frame Status Conversion1/1
  Unbuffer1/1 -> Out1/1

== system qpskTest/Subsystem24/tostring2 ==
  In1 : Inport
  In2 : Inport  Port=2
  Frame Status Conversion2 : dspobslib/Frame Status Conversion  growRefPort=off  outframe=Sample-based
      settings: SourceProductName=DSP System Toolbox  SourceProductBaseCode=DS
  Frame Status Conversion3 : dspobslib/Frame Status Conversion  growRefPort=off  outframe=Sample-based
      settings: SourceProductName=DSP System Toolbox  SourceProductBaseCode=DS
  Unbuffer2 : Unbuffer
  Unbuffer3 : Unbuffer
  Out1 : Outport
  Out2 : Outport  Port=2
  wires:
  Frame Status Conversion3/1 -> Unbuffer3/1
  Frame Status Conversion2/1 -> Unbuffer2/1
  In1/1 -> Frame Status Conversion3/1
  In2/1 -> Frame Status Conversion2/1
  Unbuffer3/1 -> Out1/1
  Unbuffer2/1 -> Out2/1

== system qpskTest/Subsystem25/tostring9 ==
  In1 : Inport
  In2 : Inport  Port=2
  Frame Status Conversion2 : dspobslib/Frame Status Conversion  growRefPort=off  outframe=Sample-based
      settings: SourceProductName=DSP System Toolbox  SourceProductBaseCode=DS
  Frame Status Conversion3 : dspobslib/Frame Status Conversion  growRefPort=off  outframe=Sample-based
      settings: SourceProductName=DSP System Toolbox  SourceProductBaseCode=DS
  Unbuffer2 : Unbuffer
  Unbuffer3 : Unbuffer
  Out1 : Outport
  Out2 : Outport  Port=2
  wires:
  Frame Status Conversion3/1 -> Unbuffer3/1
  Frame Status Conversion2/1 -> Unbuffer2/1
  In1/1 -> Frame Status Conversion3/1
  In2/1 -> Frame Status Conversion2/1
  Unbuffer3/1 -> Out1/1
  Unbuffer2/1 -> Out2/1

== system qpskTest/Subsystem26/tostring9 ==
  In1 : Inport
  In2 : Inport  Port=2
  Frame Status Conversion2 : dspobslib/Frame Status Conversion  growRefPort=off  outframe=Sample-based
      settings: SourceProductName=DSP System Toolbox  SourceProductBaseCode=DS
  Frame Status Conversion3 : dspobslib/Frame Status Conversion  growRefPort=off  outframe=Sample-based
      settings: SourceProductName=DSP System Toolbox  SourceProductBaseCode=DS
  Unbuffer2 : Unbuffer
  Unbuffer3 : Unbuffer
  Out1 : Outport
  Out2 : Outport  Port=2
  wires:
  Frame Status Conversion3/1 -> Unbuffer3/1
  Frame Status Conversion2/1 -> Unbuffer2/1
  In1/1 -> Frame Status Conversion3/1
  In2/1 -> Frame Status Conversion2/1
  Unbuffer3/1 -> Out1/1
  Unbuffer2/1 -> Out2/1

== system qpskTest/Subsystem5/Subsystem ==
  In1 : Inport
  Enable : EnablePort
  Math Function : Math  Operator=reciprocal  SaturateOnIntegerOverflow=on
  Out1 : Outport
  wires:
  In1/1 -> Math Function/1
  Math Function/1 -> Out1/1

== system qpskTest/Subsystem5/Subsystem16 ==
  In1 : Inport
  In2 : Inport  Port=2
  Complex to Real-Imag5 : ComplexToRealImag
  Complex to Real-Imag6 : ComplexToRealImag
  Scope6 : Scope  NumInputPorts=4
  tostring8 : Subsystem
  wires:
  tostring8/1(Out1) -> Scope6/1
  tostring8/2(Out2) -> Scope6/2
  Complex to Real-Imag5/1 -> tostring8/1(In1)
  Complex to Real-Imag5/2 -> tostring8/2(In2)
  Complex to Real-Imag6/1 -> tostring8/3(In3)
  Complex to Real-Imag6/2 -> tostring8/4(In4)
  tostring8/3(Out3) -> Scope6/3
  tostring8/4(Out4) -> Scope6/4
  In1/1 -> Complex to Real-Imag5/1
  In2/1 -> Complex to Real-Imag6/1

== system qpskTest/Subsystem5/Subsystem4 ==
  Enable : EnablePort
  Frame Status Conversion2 : dspobslib/Frame Status Conversion  growRefPort=off  outframe=Frame-based
      settings: SourceProductName=DSP System Toolbox  SourceProductBaseCode=DS
  Math Function : Math  Operator=reciprocal  SaturateOnIntegerOverflow=on
  PN Sequence Generator : commseqgen2/PN Sequence Generator  poly=[1 0 0 0 0 1 1]  ini_sta=[0 0 0 0 0 1]  outBitMaskSource=Dialog parameter  shift=0  outVarSiz=off  maxOutSizeMode=Dialog parameter  maxOutSize=[10 1]  Ts=16e-5/2/31  frameBased=on  sampPerFrame=31  reset=off  bitPackedOutputs=off  outDataType=double  numPackedBits=8  bitPackDataSigned=off  bitPackedOutDType=double
      settings: SourceProductName=Communications Toolbox  SourceProductBaseCode=CM
  Subsystem23 : Subsystem
  Unipolar to Bipolar Converter : commutil2/Unipolar to Bipolar Converter  M=2  polarity=Positive  dataType=Inherit via internal rule
      settings: SourceProductName=Communications Toolbox
  Out1 : Outport
  wires:
  PN Sequence Generator/1 -> Unipolar to Bipolar Converter/1
  Frame Status Conversion2/1 -> Out1/1
  Math Function/1 -> Frame Status Conversion2/1, Subsystem23/1(In1)
  Unipolar to Bipolar Converter/1 -> Math Function/1, Subsystem23/2(In2)

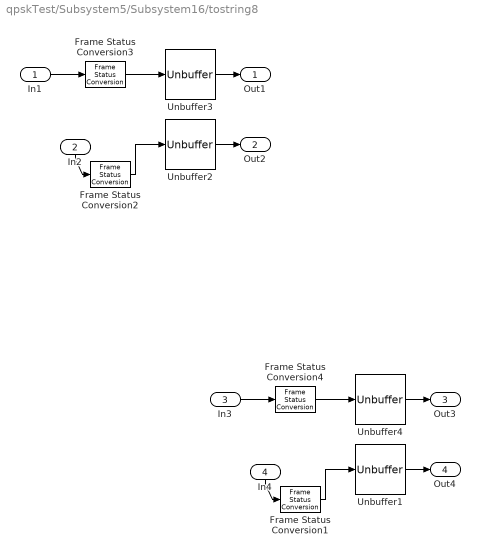
== system qpskTest/Subsystem5/Subsystem16/tostring8 ==
  In1 : Inport
  In2 : Inport  Port=2
  In3 : Inport  Port=3
  In4 : Inport  Port=4
  Frame Status Conversion{1..4} (4 alike) : dspobslib/Frame Status Conversion  growRefPort=off  outframe=Sample-based
      settings: SourceProductName=DSP System Toolbox  SourceProductBaseCode=DS
  Unbuffer{1..4} (4 alike) : Unbuffer
  Out1 : Outport
  Out2 : Outport  Port=2
  Out3 : Outport  Port=3
  Out4 : Outport  Port=4
  wires:
  Frame Status Conversion3/1 -> Unbuffer3/1
  Frame Status Conversion2/1 -> Unbuffer2/1
  In1/1 -> Frame Status Conversion3/1
  In2/1 -> Frame Status Conversion2/1
  Unbuffer3/1 -> Out1/1
  Unbuffer2/1 -> Out2/1
  Frame Status Conversion4/1 -> Unbuffer4/1
  Frame Status Conversion1/1 -> Unbuffer1/1
  In3/1 -> Frame Status Conversion4/1
  In4/1 -> Frame Status Conversion1/1
  Unbuffer4/1 -> Out3/1
  Unbuffer1/1 -> Out4/1

== system qpskTest/Subsystem5/Subsystem4/Subsystem23 ==
  In1 : Inport
  In2 : Inport  Port=2
  Scope : Scope  NumInputPorts=2
  tostring : Subsystem
  tostring1 : Subsystem
  wires:
  tostring/1(Out1) -> Scope/1
  tostring1/1(Out1) -> Scope/2
  In1/1 -> tostring/1(In1)
  In2/1 -> tostring1/1(In1)

== system qpskTest/Subsystem5/Subsystem4/Subsystem23/tostring ==
  In1 : Inport
  Frame Status Conversion5 : dspobslib/Frame Status Conversion  growRefPort=off  outframe=Sample-based
      settings: SourceProductName=DSP System Toolbox  SourceProductBaseCode=DS
  Unbuffer : Unbuffer
  Out1 : Outport
  wires:
  Frame Status Conversion5/1 -> Unbuffer/1
  In1/1 -> Frame Status Conversion5/1
  Unbuffer/1 -> Out1/1

== system qpskTest/Subsystem5/Subsystem4/Subsystem23/tostring1 ==
  In1 : Inport
  Frame Status Conversion1 : dspobslib/Frame Status Conversion  growRefPort=off  outframe=Sample-based
      settings: SourceProductName=DSP System Toolbox  SourceProductBaseCode=DS
  Unbuffer1 : Unbuffer
  Out1 : Outport
  wires:
  Frame Status Conversion1/1 -> Unbuffer1/1
  In1/1 -> Frame Status Conversion1/1
  Unbuffer1/1 -> Out1/1
